simulink model "Design_of_an_Energy_Efficient_Hybrid_Electric_Vehicle"  (R2023a)
settings: Solver=FixedStepDiscrete  StartTime=0  StopTime=110  RelTol=1e-3  EnableMultiTasking=on
PreLoadFcn:
  | power_motordrive_IPMSM_FOC_data
InitFcn:
  | power_motordrive_IPMSM_FOC_data
  | Cdc  = 0.001;      % DC-link capacitor  [F]
  | AH0  = 280;        % Initial battery charge [hr*A]
  | Tmax=410;
  | 
  | %% Vehicle Parameters for Vehicle Dynamics 2
  | vehicle_mass = 2111;
  | wheel_radius = 0.228;
  | area =2.22;
  | drag_coefficient = 0.23;
  | air_density = 1.204;
  | gravity = 9.81;
  | rolling_res_ratio = 0.02;
  | 
  | % Differential drive parameters
  | gear_ratio = 5;
  | i_t   = gear_ratio ;
  | Rw=wheel_radius;
  | 
  | 
  | %% Sliding Mode Observer
  | pmsm.N_max=wmax;
  | pmsm.p=p
  | pmsm.Ld=Ld;
  | pmsm.Lq=Lq;
  | pmsm.Rs=Rs;
  | PU_System.V_base=(Vdc_nom/sqrt(3));
  | PU_System.I_base=lambda/(Lq-Ld);
  | max_torque=400
  | force_max_pedal=500
  | braking_torque_to_pedal_force_ratio=-4
undefined symbols (not defined in the file): BlkSampleTime, CurrentObserverGain, dataType, DiscIntNeverNeededParam, Fsw, gcbh, Ki_Ireg, Ki_wreg, Kp_Ireg, Kp_wreg, L_smo_gain, lambda, Ld, Limit_Ireg, Limit_wreg, Lq, MaxApplicationSpeed, MaxStatorCurrent, MaxStatorVoltage, NumBits1, NumBits2, p, Pmsm, PolePairs, QPLL, rpm_data, Sensorless, sigbuilder_block, SlidingLimit, Slope1, Slope2, sps_rtmsupport, StatorInductance, StatorResistance, Tmax_data, Tnom, Ts, Vdc_nom, wmax
libraries: fl_lib x27, nesl_utility x24, simulink x23, mcbcontrolslib x15, fl_ps_legacy_lib x9, spsStairGeneratorLib x7, sdl_lib x6, ee_lib x4, mcbpositiondecoderlib x4, BoomBox x3, tiiqmathlib x2, autolibshared x2
(part 2 of 4)

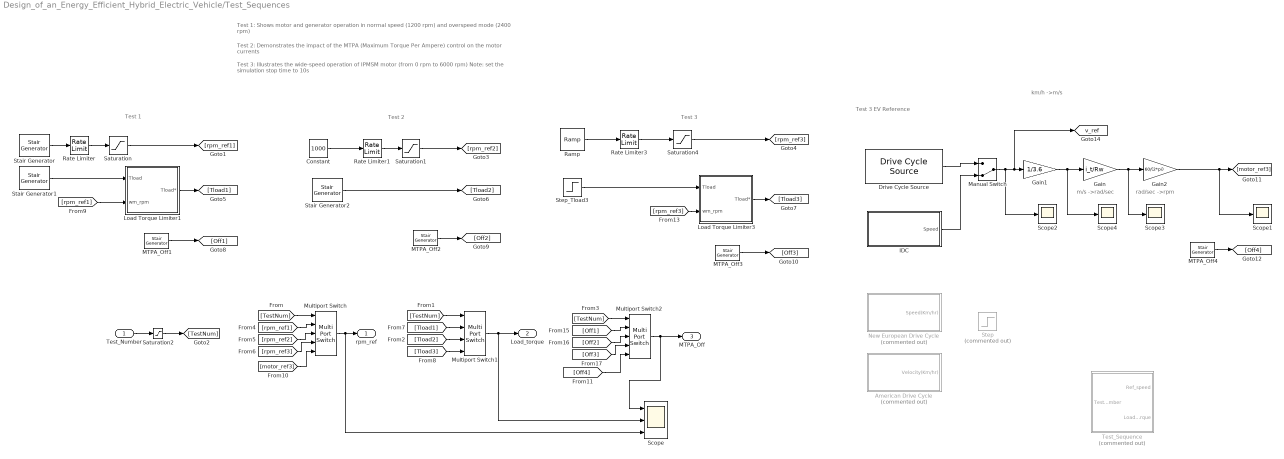
== system Design_of_an_Energy_Efficient_Hybrid_Electric_Vehicle/Test_Sequences ==
  note: Test 1
  note: Test 2
  note: Test 3
  note: Test 1: Shows motor and generator operation in normal speed (1200 rpm) and overspeed mode (2400 rpm)
  note: Test 2: Demonstrates the impact of the MTPA (Maximum Torque Per Ampere) control on the motor currents
  note: Test 3: Illustrates the wide-speed operation of IPMSM motor (from 0 rpm to 6000 rpm)
      | Note: set the simulation stop time to 10s
  note: Test 3 EV Reference
  note: rad/sec ->rpm
  note: m/s ->rad/sec
  note: km/h ->m/s
  Test_Number : Inport
  American Drive Cycle : Subsystem  Tag=STV Subsys  Commented=on  LoadFcn=sigbuilder_block('load');  StartFcn=sigbuilder_block('start');  StopFcn=sigbuilder_block('stop');  ClipboardFcn=sigbuilder_block('clipboard');  mask(Sigbuilder block){tuvar=[0:10]}
      mask help: Simulink:masks:SigbuilderBlock_MD
      mask init:
      | if ~strcmp(get_param(bdroot(gcbh),'SimulationStatus'),'stopped') tuvar = sigbuilder_block('maskInit'); end
      settings: CopyFcn=sigbuilder_block('copy');  DeleteFcn=sigbuilder_block('delete');  ModelCloseFcn=sigbuilder_block('modelClose');  PreSaveFcn=sigbuilder_block('preSave');  PauseFcn=sigbuilder_block('pause');  ContinueFcn=sigbuilder_block('continue');  NameChangeFcn=sigbuilder_block('namechange');  OpenFcn=sigbuilder_block('open',[423.6 162.6 550.8 400.2 ]);  CloseFcn=sigbuilder_block('close');
      mask Display: plot(0, 0, 100, 100,[2, 2, 32, 32, 2], [68, 8, 8, 68, 68],[32, 2], [38, 38], [32, 19, 2],[53, 60, 44], [32, 17, 17, 2],[16, 16, 31, 31]);txt = getActiveGroup(gcbh);text(2, 100, txt,'verticalAlignment', 'top');
  Constant : Constant  Value=1000
  Drive Cycle Source : autolibshared/Drive Cycle Source  cycleVar=FTP75  fileVar=cycleFTP75.mat  tfinal="2474  seconds"  cycleRepeat=off  outAccPort=off  outGearPort=off  gearList=No gear data  t_wot1=5  xdot_woto=0  xdot_wot1=30  t_wot2=20  xdot_wot2=0  t_wotend=30  srcUnit=m/s  outUnit=km/h  srcAccUnit=m/s/s  outAccUnit=m/s^2  dt=0  aMode=1  faultOption=off  velBnd=2  velBndUnit=mph  inUnit=m/s  timeBnd=1  failOption=off  stopSim=off  maxFaultCnt=10  maxFaultTime=2  maxTotFaultTime=15  traceOption=off  dtTrace=1  traceWindow=10  lastDCname=FTP75  lastOutUnit=mph  lastDT=0  lastTB=1  lastSB=2  forceCalcBound=off
  Gain : Gain  Gain=i_t/Rw
  Gain1 : Gain  Gain=1/3.6
  Gain2 : Gain  Gain=60/(2*pi)
  IDC : Subsystem  Tag=STV Subsys  LoadFcn=sigbuilder_block('load');  StartFcn=sigbuilder_block('start');  StopFcn=sigbuilder_block('stop');  ClipboardFcn=sigbuilder_block('clipboard');  mask(Sigbuilder block){tuvar=[0:10]}
      mask help: Simulink:masks:SigbuilderBlock_MD
      mask init:
      | if ~strcmp(get_param(bdroot(gcbh),'SimulationStatus'),'stopped') tuvar = sigbuilder_block('maskInit'); end
      settings: CopyFcn=sigbuilder_block('copy');  DeleteFcn=sigbuilder_block('delete');  ModelCloseFcn=sigbuilder_block('modelClose');  PreSaveFcn=sigbuilder_block('preSave');  PauseFcn=sigbuilder_block('pause');  ContinueFcn=sigbuilder_block('continue');  NameChangeFcn=sigbuilder_block('namechange');  OpenFcn=sigbuilder_block('open',[441 202.5 577.5 270 ]);  CloseFcn=sigbuilder_block('close');
      mask Display: plot(0, 0, 100, 100,[2, 2, 32, 32, 2], [68, 8, 8, 68, 68],[32, 2], [38, 38], [32, 19, 2],[53, 60, 44], [32, 17, 17, 2],[16, 16, 31, 31]);txt = getActiveGroup(gcbh);text(2, 100, txt,'verticalAlignment', 'top');
  Load Torque Limiter1 : Subsystem
  Load Torque Limiter3 : Subsystem
  MTPA_Off1 : spsStairGeneratorLib/Stair Generator  t=[0, 0.9]  e=[0, 1]*0  Ts=Ts
  MTPA_Off2 : spsStairGeneratorLib/Stair Generator  t=[0, 0.8]  e=[0, 1]  Ts=Ts
  MTPA_Off3 : spsStairGeneratorLib/Stair Generator  t=[0, 1.8]  e=[0, 1]*0  Ts=Ts
  MTPA_Off4 : spsStairGeneratorLib/Stair Generator  t=[0, 1.8]  e=[0, 1]*0  Ts=Ts
  Manual Switch : ManualSwitch  CurrentSetting=0
  Multiport Switch : MultiPortSwitch  Inputs=4  SaturateOnIntegerOverflow=off  InputSameDT=off
  Multiport Switch1 : MultiPortSwitch  SaturateOnIntegerOverflow=off  InputSameDT=off
  Multiport Switch2 : MultiPortSwitch  Inputs=4  SaturateOnIntegerOverflow=off  InputSameDT=off
  New European Drive Cycle : Subsystem  Tag=STV Subsys  Commented=on  LoadFcn=sigbuilder_block('load');  StartFcn=sigbuilder_block('start');  StopFcn=sigbuilder_block('stop');  ClipboardFcn=sigbuilder_block('clipboard');  mask(Sigbuilder block){tuvar=[0:10]}
      mask help: Simulink:masks:SigbuilderBlock_MD
      mask init:
      | if ~strcmp(get_param(bdroot(gcbh),'SimulationStatus'),'stopped') tuvar = sigbuilder_block('maskInit'); end
      settings: CopyFcn=sigbuilder_block('copy');  DeleteFcn=sigbuilder_block('delete');  ModelCloseFcn=sigbuilder_block('modelClose');  PreSaveFcn=sigbuilder_block('preSave');  PauseFcn=sigbuilder_block('pause');  ContinueFcn=sigbuilder_block('continue');  NameChangeFcn=sigbuilder_block('namechange');  OpenFcn=sigbuilder_block('open',[75.6 -6 550.8 400.2 ]);  CloseFcn=sigbuilder_block('close');
      mask Display: plot(0, 0, 100, 100,[2, 2, 32, 32, 2], [68, 8, 8, 68, 68],[32, 2], [38, 38], [32, 19, 2],[53, 60, 44], [32, 17, 17, 2],[16, 16, 31, 31]);txt = getActiveGroup(gcbh);text(2, 100, txt,'verticalAlignment', 'top');
  Ramp : simulink/Sources/Ramp  slope=1000*0.7  start=0.5  InitialOutput=0
  Rate Limiter : RateLimiter  RisingSlewLimit=8000  FallingSlewLimit=-8000  SampleTimeMode=inherited
  Rate Limiter1 : RateLimiter  RisingSlewLimit=10000  FallingSlewLimit=-10000  SampleTimeMode=inherited
  Rate Limiter3 : RateLimiter  RisingSlewLimit=5000  FallingSlewLimit=-5000  SampleTimeMode=inherited
  Saturation : Saturate  UpperLimit=wmax  LowerLimit=0
  Saturation1 : Saturate  UpperLimit=wmax  LowerLimit=0
  Saturation2 : Saturate  UpperLimit=4  LowerLimit=1
  Saturation4 : Saturate  UpperLimit=wmax  LowerLimit=0
  Scope : Scope  NumInputPorts=3
  Scope{1..4} (4 alike) : Scope
  Stair Generator : spsStairGeneratorLib/Stair Generator  t=[0,0.7]  e=[1200,2400]  Ts=Ts
  Stair Generator1 : spsStairGeneratorLib/Stair Generator  t="[0,0.4,0.7  1]"  e=[0, 350, 150 -150]  Ts=Ts
  Stair Generator2 : spsStairGeneratorLib/Stair Generator  t=[0,0.4]  e=[0, 350 ]  Ts=Ts
  Step : Step  Commented=on  After=30
  Step_Tload3 : Step  Before=1  After=Tnom  SampleTime=Ts
  Test_Sequence : Subsystem  Commented=on
  rpm_ref : Outport
  Load_torque : Outport  Port=2
  MTPA_Off : Outport  Port=3
  tag scope: v_ref=global
  wires:
  Stair Generator/1 -> Rate Limiter/1
  Rate Limiter/1 -> Saturation/1
  Saturation/1 -> [rpm_ref1]
  Multiport Switch/1 -> Scope/3, rpm_ref/1
  Test_Number/1 -> Saturation2/1
  Saturation2/1 -> [TestNum]
  [TestNum] -> Multiport Switch/1
  Rate Limiter3/1 -> Saturation4/1
  Saturation4/1 -> [rpm_ref3]
  [rpm_ref1] -> Multiport Switch/2
  [rpm_ref2] -> Multiport Switch/3
  [rpm_ref3] -> Multiport Switch/4
  [Tload3] -> Multiport Switch1/4
  [Tload2] -> Multiport Switch1/3
  [Tload1] -> Multiport Switch1/2
  [TestNum] -> Multiport Switch1/1
  Multiport Switch1/1 -> Scope/2, Load_torque/1
  Load Torque Limiter3/1(Tload*) -> [Tload3]
  Multiport Switch2/1 -> Scope/1, MTPA_Off/1
  [TestNum] -> Multiport Switch2/1
  [Off1] -> Multiport Switch2/2
  [Off2] -> Multiport Switch2/3
  [Off3] -> Multiport Switch2/4
  MTPA_Off1/1 -> [Off1]
  MTPA_Off2/1 -> [Off2]
  MTPA_Off3/1 -> [Off3]
  Saturation1/1 -> [rpm_ref2]
  Rate Limiter1/1 -> Saturation1/1
  Constant/1 -> Rate Limiter1/1
  Ramp/1 -> Rate Limiter3/1
  [rpm_ref3] -> Load Torque Limiter3/2(wm_rpm)
  [rpm_ref1] -> Load Torque Limiter1/2(wm_rpm)
  Load Torque Limiter1/1(Tload*) -> [Tload1]
  Step_Tload3/1 -> Load Torque Limiter3/1(Tload)
  Stair Generator1/1 -> Load Torque Limiter1/1(Tload)
  Stair Generator2/1 -> [Tload2]
  Drive Cycle Source/1 -> Manual Switch/1
  Gain1/1 -> Scope4/1, Gain/1
  Gain2/1 -> Scope1/1, [motor_ref3]
  Gain/1 -> Scope3/1, Gain2/1
  [motor_ref3] -> Multiport Switch/5
  MTPA_Off4/1 -> [Off4]
  [Off4] -> Multiport Switch2/5
  Manual Switch/1 -> Scope2/1, [v_ref], Gain1/1
  IDC/1(Speed) -> Manual Switch/2

== system Design_of_an_Energy_Efficient_Hybrid_Electric_Vehicle/Vehicle Controller ==
  Acc : Inport
  Brk : Inport  Port=2
  Rate Transition : RateTransition
  Rate Transition1 : RateTransition
  Rate Transition2 : RateTransition
  Task_10ms : simulink/Ports & Subsystems/Function-Call Generator  sample_time=0.01  numberOfIterations=1  DisallowWideOutput=off
  Vehicle Controller : Subsystem
  trqR : Outport  VectorParamsAs1DForOutWhenUnconnected=off
  tag scope: Acceleration=global, Brake=global
  wires:
  Acc/1 -> Rate Transition/1
  Task_10ms/1 -> Vehicle Controller/Trigger
  Vehicle Controller/1(TqRequest) -> trqR/1
  Brk/1 -> Rate Transition1/1
  Rate Transition/1 -> Vehicle Controller/1(AccPedal [0,1]), [Acceleration]
  Rate Transition1/1 -> [Brake], Vehicle Controller/2(BrakePedal [0,1])
  [v] -> Rate Transition2/1
  Rate Transition2/1 -> Vehicle Controller/3(v [km/h])

== system Design_of_an_Energy_Efficient_Hybrid_Electric_Vehicle/All-Terrain Vehicle Model/Brake Torque ==
  Pedal : Inport
  Dead Zone : DeadZone  LowerValue=-Tmax*i_t  UpperValue=Tmax*i_t
  Force for max pedal deflection : Gain  Gain=force_max_pedal
  Ideal Torque Source : fl_lib/Mechanical/Mechanical Sources/Ideal Torque Source
  MRRef : fl_lib/Mechanical/Rotational Elements/Mechanical Rotational Reference
  Motion Sensor : fl_lib/Mechanical/Mechanical Sensors/Ideal Rotational Motion Sensor  reference=foundation.enum.MeasurementReference.difference  acceleration_port=false  velocity_port=true  position_port=true  wrap_angle=simscape.enum.onoff.off  offset=0 rad
  PS Product : fl_ps_legacy_lib/Legacy Physical Signals/Functions/PS Product
  Scope : Scope
  Scope1 : Scope
  Scope2 : Scope
  Simulink-PS Converter1 : nesl_utility/Simulink-PS Converter  PhysicalDomain=network_engine_domain  SubClassName=ps_input  LeftPortType=input  RightPortType=output  PseudoPeriodic=off  Frequencies=[]  NoiseDistribution=none  NoiseParameters=[]  Unit=N*m  AffineConversion=off  FilteringAndDerivatives=zero  SimscapeFilterOrder=1  InputFilterTimeConstant=0.001  UdotUserProvided=1
  Smooth Sign : Subsystem
  Torque per unit brake pedal force : Gain  Gain=braking_torque_to_pedal_force_ratio
  R : PMIOPort  Side=Right
  wires:
  Pedal/1 -> Force for max pedal deflection/1
  Force for max pedal deflection/1 -> Scope2/1, Torque per unit brake pedal force/1
  Torque per unit brake pedal force/1 -> Scope/1, Dead Zone/1
  Dead Zone/1 -> Scope1/1, Simulink-PS Converter1/1
  connections:
  Smooth Sign/RConn1 -- PS Product/LConn2
  Motion Sensor/RConn1 -- MRRef/LConn1 -- Ideal Torque Source/RConn2
  Ideal Torque Source/LConn1 -- Motion Sensor/LConn1 -- R/RConn1
  PS Product/RConn1 -- Ideal Torque Source/RConn1
  Simulink-PS Converter1/RConn1 -- PS Product/LConn1
  Smooth Sign/LConn1 -- Motion Sensor/RConn2

== system Design_of_an_Energy_Efficient_Hybrid_Electric_Vehicle/All-Terrain Vehicle Model/Sensor Subsystem ==
  Ideal Translational Motion Sensor : fl_lib/Mechanical/Mechanical Sensors/Ideal Translational Motion Sensor  reference=foundation.enum.MeasurementReference.difference  acceleration_port=false  velocity_port=true  position_port=true  offset=0 m
  Mechanical Translational Reference : fl_lib/Mechanical/Translational Elements/Mechanical Translational Reference
  PS-Simulink Converter1 : nesl_utility/PS-Simulink Converter  PhysicalDomain=network_engine_domain  SubClassName=ps_output  LeftPortType=input  RightPortType=output  PseudoPeriodic=off  Frequencies=[]  VectorFormat=1-D array  Unit=km/hr  AffineConversion=off
  PS-Simulink Converter2 : nesl_utility/PS-Simulink Converter  PhysicalDomain=network_engine_domain  SubClassName=ps_output  LeftPortType=input  RightPortType=output  PseudoPeriodic=off  Frequencies=[]  VectorFormat=1-D array  Unit=1  AffineConversion=off
  PS-Simulink Converter3 : nesl_utility/PS-Simulink Converter  PhysicalDomain=network_engine_domain  SubClassName=ps_output  LeftPortType=input  RightPortType=output  PseudoPeriodic=off  Frequencies=[]  VectorFormat=1-D array  Unit=mph  AffineConversion=off
  Vehicle : PMIOPort  Side=Left
  Pos : PMIOPort  Port=2  Side=Right
  mph : Outport  VectorParamsAs1DForOutWhenUnconnected=off
  kmph : Outport  Port=2  VectorParamsAs1DForOutWhenUnconnected=off
  m : Outport  Port=3  VectorParamsAs1DForOutWhenUnconnected=off
  wires:
  PS-Simulink Converter1/1 -> kmph/1
  PS-Simulink Converter2/1 -> m/1
  PS-Simulink Converter3/1 -> mph/1
  connections:
  Mechanical Translational Reference/LConn1 -- Ideal Translational Motion Sensor/RConn1
  PS-Simulink Converter2/LConn1 -- Pos/RConn1 -- Ideal Translational Motion Sensor/RConn3
  Ideal Translational Motion Sensor/RConn2 -- PS-Simulink Converter3/LConn1 -- PS-Simulink Converter1/LConn1
  Ideal Translational Motion Sensor/LConn1 -- Vehicle/RConn1

== system Design_of_an_Energy_Efficient_Hybrid_Electric_Vehicle/Electric Drive/Gate Driver ==
  S : Inport
  Demux : Demux  Outputs=6
  Simulink-PS Converter{1..6} (6 alike) : nesl_utility/Simulink-PS Converter  PhysicalDomain=network_engine_domain  SubClassName=ps_input  LeftPortType=input  RightPortType=output  PseudoPeriodic=off  Frequencies=[]  NoiseDistribution=none  NoiseParameters=[]  Unit=1  AffineConversion=off  FilteringAndDerivatives=zero  SimscapeFilterOrder=1  InputFilterTimeConstant=0.001  UdotUserProvided=1
  Six-Pulse Gate Multiplexer : ee_lib/Semiconductors & Converters/Converters/Six-Pulse Gate Multiplexer  port_option=ee.enum.controlport.ps
  G : PMIOPort  Side=Right
  wires:
  Demux/1 -> Simulink-PS Converter1/1
  S/1 -> Demux/1
  Demux/4 -> Simulink-PS Converter4/1
  Demux/2 -> Simulink-PS Converter2/1
  Demux/3 -> Simulink-PS Converter3/1
  Demux/5 -> Simulink-PS Converter5/1
  Demux/6 -> Simulink-PS Converter6/1
  connections:
  Six-Pulse Gate Multiplexer/RConn1 -- G/RConn1
  Simulink-PS Converter1/RConn1 -- Six-Pulse Gate Multiplexer/LConn1
  Simulink-PS Converter3/RConn1 -- Six-Pulse Gate Multiplexer/LConn3
  Simulink-PS Converter5/RConn1 -- Six-Pulse Gate Multiplexer/LConn5
  Simulink-PS Converter6/RConn1 -- Six-Pulse Gate Multiplexer/LConn6
  Simulink-PS Converter4/RConn1 -- Six-Pulse Gate Multiplexer/LConn4
  Simulink-PS Converter2/RConn1 -- Six-Pulse Gate Multiplexer/LConn2

== system Design_of_an_Energy_Efficient_Hybrid_Electric_Vehicle/Electric Drive/Meas I ==
  Current Sensor : ee_lib/Sensors & Transducers/Current Sensor (Three-Phase)
  PS-Simulink Converter : nesl_utility/PS-Simulink Converter  PhysicalDomain=network_engine_domain  SubClassName=ps_output  LeftPortType=input  RightPortType=output  PseudoPeriodic=off  Frequencies=[]  VectorFormat=1-D array  Unit=A  AffineConversion=off
  1 : PMIOPort  Side=Left
  2 : PMIOPort  Port=2  Side=Right
  iabc : Outport  VectorParamsAs1DForOutWhenUnconnected=off
  tag scope: I_ABC=global
  wires:
  PS-Simulink Converter/1 -> [I_ABC], iabc/1
  connections:
  1/RConn1 -- Current Sensor/LConn1
  2/RConn1 -- Current Sensor/RConn2
  Current Sensor/RConn1 -- PS-Simulink Converter/LConn1

== system Design_of_an_Energy_Efficient_Hybrid_Electric_Vehicle/Electric Drive/Meas V ==
  PS-Simulink Converter4 : nesl_utility/PS-Simulink Converter  PhysicalDomain=network_engine_domain  SubClassName=ps_output  LeftPortType=input  RightPortType=output  PseudoPeriodic=off  Frequencies=[]  VectorFormat=1-D array  Unit=V  AffineConversion=off
  Voltage Sensor : fl_lib/Electrical/Electrical Sensors/Voltage Sensor
  - : PMIOPort  Side=Right
  + : PMIOPort  Port=2  Side=Left
  Vdc : Outport  VectorParamsAs1DForOutWhenUnconnected=off
  wires:
  PS-Simulink Converter4/1 -> Vdc/1
  connections:
  PS-Simulink Converter4/LConn1 -- Voltage Sensor/RConn1
  Voltage Sensor/LConn1 -- +/RConn1
  Voltage Sensor/RConn2 -- -/RConn1

== system Design_of_an_Energy_Efficient_Hybrid_Electric_Vehicle/Electric Drive/Sensor ==
  Display : Display
  Gain : Gain  Gain=30/pi
  MRRef : fl_lib/Mechanical/Rotational Elements/Mechanical Rotational Reference
  Motion Sensor : fl_lib/Mechanical/Mechanical Sensors/Ideal Rotational Motion Sensor  reference=foundation.enum.MeasurementReference.difference  acceleration_port=false  velocity_port=true  position_port=true  wrap_angle=simscape.enum.onoff.off  offset=0 deg
  PS-Simulink Converter1 : nesl_utility/PS-Simulink Converter  PhysicalDomain=network_engine_domain  SubClassName=ps_output  LeftPortType=input  RightPortType=output  PseudoPeriodic=off  Frequencies=[]  VectorFormat=1-D array  Unit=rad/s  AffineConversion=off
  PS-Simulink Converter2 : nesl_utility/PS-Simulink Converter  PhysicalDomain=network_engine_domain  SubClassName=ps_output  LeftPortType=input  RightPortType=output  PseudoPeriodic=off  Frequencies=[]  VectorFormat=1-D array  Unit=rad  AffineConversion=off
  PS-Simulink Converter3 : nesl_utility/PS-Simulink Converter  PhysicalDomain=network_engine_domain  SubClassName=ps_output  LeftPortType=input  RightPortType=output  PseudoPeriodic=off  Frequencies=[]  VectorFormat=1-D array  Unit=N*m  AffineConversion=off
  Scope : Scope
  Scope1 : Scope
  Torque Sensor : fl_lib/Mechanical/Mechanical Sensors/Ideal Torque Sensor
  R : PMIOPort  Side=Left
  C : PMIOPort  Port=2  Side=Right
  w : Outport  VectorParamsAs1DForOutWhenUnconnected=off
  A : Outport  Port=2  VectorParamsAs1DForOutWhenUnconnected=off
  tag scope: Tq_meas=global
  wires:
  PS-Simulink Converter1/1 -> Gain/1, w/1
  PS-Simulink Converter2/1 -> A/1
  PS-Simulink Converter3/1 -> Scope/1, [Tq_meas]
  Gain/1 -> Display/1, Scope1/1
  connections:
  Motion Sensor/RConn2 -- PS-Simulink Converter1/LConn1
  Motion Sensor/RConn1 -- MRRef/LConn1
  R/RConn1 -- Torque Sensor/LConn1
  Torque Sensor/RConn1 -- C/RConn1 -- Motion Sensor/LConn1
  Torque Sensor/RConn2 -- PS-Simulink Converter3/LConn1
  Motion Sensor/RConn3 -- PS-Simulink Converter2/LConn1

== system Design_of_an_Energy_Efficient_Hybrid_Electric_Vehicle/FOC/Alpha&Beta Current Estimation ==
  theta : Inport
  Idq_ref : Inport  Port=2
  Alpha_Beta_Estimation : Subsystem
  Scope6 : Scope
  Transfrom_Alpha_Beta_Estimation : Subsystem
  Ialpha_est : Outport
  Ibeta_est : Outport  Port=2
  "Ialpha\"_est" : Outport  Port=3
  "Ibeta\"_est" : Outport  Port=4
  wires:
  Alpha_Beta_Estimation/1(Ialpha_est) -> Ialpha_est/1
  Idq_ref/1 -> Scope6/1, Alpha_Beta_Estimation/1(Idq_ref), Transfrom_Alpha_Beta_Estimation/1(Idq_ref)
  theta/1 -> Transfrom_Alpha_Beta_Estimation/2(theta), Alpha_Beta_Estimation/2(Theta)
  Alpha_Beta_Estimation/2(Ibeta_est) -> Ibeta_est/1
  Transfrom_Alpha_Beta_Estimation/1("Ialpha\"_est") -> "Ialpha\"_est"/1
  Transfrom_Alpha_Beta_Estimation/2("Ibeta\"_est") -> "Ibeta\"_est"/1

== system Design_of_an_Energy_Efficient_Hybrid_Electric_Vehicle/FOC/Axis Transformation ==
  a : Inport
  b : Inport  Port=2
  -one_by_sqrt3 : Gain  Gain=-1/sqrt(3)  RndMeth=Simplest  OutDataTypeStr=Inherit: Same as input
  a_plus_2b : Sum  Inputs=+++  RndMeth=Simplest  OutDataTypeStr=Inherit: Same as first input
  "Alpha\"" : Outport  VectorParamsAs1DForOutWhenUnconnected=off
  "Beta\"" : Outport  Port=2  VectorParamsAs1DForOutWhenUnconnected=off
  wires:
  a_plus_2b/1 -> -one_by_sqrt3/1
  b/1 -> "Alpha\""/1, a_plus_2b/3
  -one_by_sqrt3/1 -> "Beta\""/1
  a/1 -> a_plus_2b/2, a_plus_2b/1

== system Design_of_an_Energy_Efficient_Hybrid_Electric_Vehicle/FOC/Current reference calculation ==
  Tref : Inport
  wm : Inport  Port=2
  Abs : Abs  SaturateOnIntegerOverflow=off
  Gain1 : Gain  Gain=pi/30
  Gain2 : Gain  Gain=1/Teb  SaturateOnIntegerOverflow=on  OutDataTypeStr=Inherit: Same as input  ParamDataTypeStr=Inherit: Same as input
  Gain3 : Gain  Gain=ib  SaturateOnIntegerOverflow=on  OutDataTypeStr=Inherit: Same as input  ParamDataTypeStr=Inherit: Same as input
  Gain4 : Gain  Gain=ib  SaturateOnIntegerOverflow=on  OutDataTypeStr=Inherit: Same as input  ParamDataTypeStr=Inherit: Same as input
  Ld Lq lam p ib : Constant  Value=[Ld, Lq, lam, p, lam/(Lq-Ld)]
  Ld Lq lam p ib1 : Constant  Value=lam/(Lq-Ld)
  MTPA Field Weakening Controller : MATLAB Function  TreatAsAtomicUnit=on  SystemSampleTime=Ts
  Mux : Mux  Inputs=2
  Optimal iqn : Lookup  InputValues=ten  Table=iqn  SaturateOnIntegerOverflow=off
  Rate Limiter1 : RateLimiter  RisingSlewLimit=20  FallingSlewLimit=-20  SampleTimeMode=inherited
  Rate Limiter4 : RateLimiter  RisingSlewLimit=20*5  FallingSlewLimit=-20*5  SampleTimeMode=inherited
  Scope : Scope
  Vdc : Constant  Value=Vdc_nom
  IdIq_ref : Outport
  wires:
  Mux/1 -> IdIq_ref/1
  Gain3/1 -> Mux/2
  Gain4/1 -> Mux/1
  Tref/1 -> Gain2/1
  Gain2/1 -> Abs/1, MTPA Field Weakening Controller/2(Ten)  "Ten"
  wm/1 -> Gain1/1
  Ld Lq lam p ib/1 -> MTPA Field Weakening Controller/5(params)
  Optimal iqn/1 -> MTPA Field Weakening Controller/1(iqn_opt)
  Abs/1 -> Optimal iqn/1
  Vdc/1 -> MTPA Field Weakening Controller/4(Vdc)
  Gain1/1 -> MTPA Field Weakening Controller/3(w)
  MTPA Field Weakening Controller/1(iqn) -> Rate Limiter4/1
  MTPA Field Weakening Controller/2(idn) -> Rate Limiter1/1
  Rate Limiter1/1 -> Gain4/1
  Rate Limiter4/1 -> Gain3/1
  Ld Lq lam p ib1/1 -> Scope/1

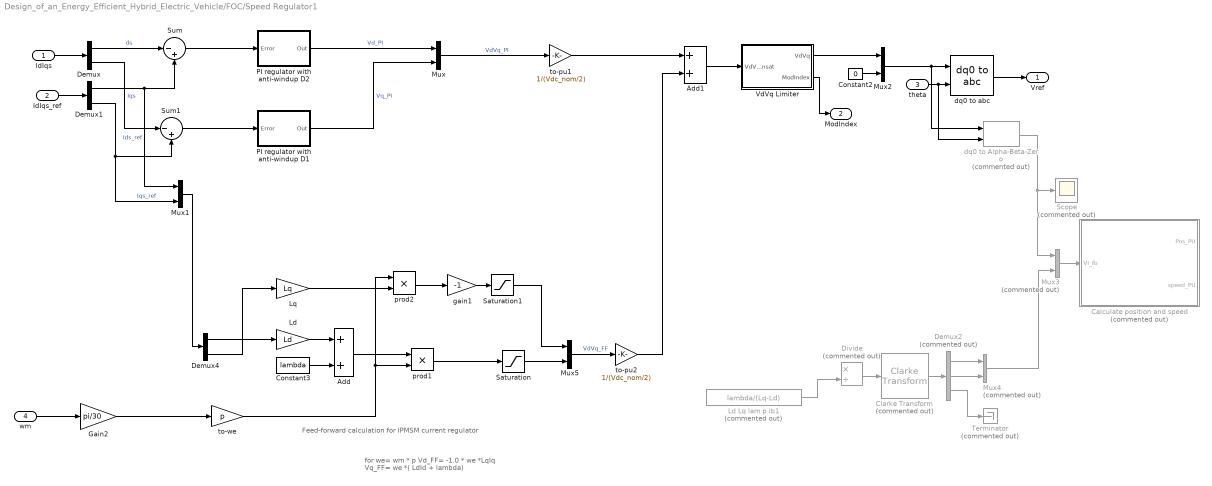
== system Design_of_an_Energy_Efficient_Hybrid_Electric_Vehicle/FOC/Speed Regulator1 ==
  note: for we= wm * p
      | Vd_FF= -1.0 * we *LqIq
      | Vq_FF= we *( LdId + lambda)
  note: Feed-forward calculation for IPMSM current regulator
  IdIqs : Inport  PortDimensions=2
  IdIqs_ref : Inport  Port=2  PortDimensions=2
  theta : Inport  Port=3  PortDimensions=1
  wm : Inport  Port=4  PortDimensions=1
  Add : Sum
  Add1 : Sum
  Calculate position and speed : Subsystem  Commented=on
  Clarke Transform : eeTransforms/Clarke Transform  Commented=on  PowerInvariant=off
  Constant2 : Constant  Value=0
  Constant3 : Constant  Value=lambda  OutDataTypeStr=Inherit: Inherit via back propagation  SampleTime=-1
  Demux : Demux  Outputs=2
  Demux1 : Demux  Outputs=2
  Demux2 : Demux  Commented=on  Outputs=3
  Demux4 : Demux  Outputs=2
  Divide : Product  Commented=on  Inputs=*/
  Gain2 : Gain  Gain=pi/30
  Ld : Gain  Gain=Ld  RndMeth=Simplest  OutDataTypeStr=Inherit: Same as input  ParamDataTypeStr=Inherit: Same as input
  Ld Lq lam p ib1 : Constant  Commented=on  Value=lambda/(Lq-Ld)
  Lq : Gain  Gain=Lq  RndMeth=Simplest  OutDataTypeStr=Inherit: Same as input  ParamDataTypeStr=Inherit: Same as input
  Mux : Mux  Inputs=2
  Mux1 : Mux  Inputs=2
  Mux2 : Mux  Inputs=[2,1]
  Mux3 : Mux  Commented=on  Inputs=2
  Mux4 : Mux  Commented=on  Inputs=2
  Mux5 : Mux  Inputs=2
  PI regulator with anti-windup D1 : Subsystem  DialogController=POWERSYS.PowerSysDialog  mask(Discrete PI Controller){Kp=Kp, Ki=Ki, Par_Limits=[Limits -Limits], Init=0, Ts=Ts}
      mask prompts: Kp "Proportional gain (Kp):"; Ki "Integral gain (Ki):"; Par_Limits "Output limits: [ Upper   Lower ]"; Init "Output initial value:"; Ts "Sample time:"
      mask help: This block implements a discrete PI controller.
      mask init:
      | UpperLimit=Par_Limits(1);
      | LowerLimit=Par_Limits(2);
      | power_initmask();
      mask Help: This block is part of a subset of blocks in the Extras library that does not have documentation associated with it, other than the block mask description.
      mask Display: disp('PI');
  PI regulator with anti-windup D2 : Subsystem  DialogController=POWERSYS.PowerSysDialog  mask(Discrete PI Controller){Kp=Kp, Ki=Ki, Par_Limits=[Limits -Limits], Init=0, Ts=Ts}
      mask prompts: Kp "Proportional gain (Kp):"; Ki "Integral gain (Ki):"; Par_Limits "Output limits: [ Upper   Lower ]"; Init "Output initial value:"; Ts "Sample time:"
      mask help: This block implements a discrete PI controller.
      mask init:
      | UpperLimit=Par_Limits(1);
      | LowerLimit=Par_Limits(2);
      | power_initmask();
      mask Help: This block is part of a subset of blocks in the Extras library that does not have documentation associated with it, other than the block mask description.
      mask Display: disp('PI');
  Saturation : Saturate  UpperLimit=Vdc_nom/sqrt(3)  LowerLimit=-Vdc_nom/sqrt(3)  RndMeth=Simplest
  Saturation1 : Saturate  UpperLimit=Vdc_nom/sqrt(3)  LowerLimit=-Vdc_nom/sqrt(3)  RndMeth=Simplest
  Scope : Scope  Commented=on
  Sum : Sum  Inputs=|-+
  Sum1 : Sum  Inputs=|-+
  Terminator : Terminator  Commented=on
  VdVq Limiter : Subsystem
  dq0 to Alpha-Beta-Zero : spsdq0toAlphaBetaZeroLib/dq0 to Alpha-Beta-Zero  Commented=on  Alignment=90 degrees behind phase A axis
  dq0 to abc : spsdq0toabcLib/dq0 to abc  Alignment=90 degrees behind phase A axis
  gain1 : Gain  Gain=-1  RndMeth=Simplest  OutDataTypeStr=Inherit: Same as input  ParamDataTypeStr=Inherit: Same as input
  prod1 : Product  RndMeth=Simplest  OutDataTypeStr=Inherit: Same as first input
  prod2 : Product  RndMeth=Simplest  OutDataTypeStr=Inherit: Same as first input
  to-pu1 : Gain  Gain=1/(Vdc_nom/2)
  to-pu2 : Gain  Gain=1/(Vdc_nom/2)
  to-we : Gain  Gain=p  RndMeth=Simplest  OutDataTypeStr=Inherit: Same as input  ParamDataTypeStr=Inherit: Same as input
  Vref : Outport
  ModIndex : Outport  Port=2
  wires:
  to-pu2/1 -> Add1/2
  to-pu1/1 -> Add1/1
  Demux1/1 -> Mux1/1, Sum/2  "Ids_ref"
  Demux/1 -> Sum/1  "ds"
  Demux1/2 -> Sum1/2, Mux1/2  "Iqs_ref"
  IdIqs_ref/1 -> Demux1/1
  IdIqs/1 -> Demux/1
  Sum/1 -> PI regulator with anti-windup D2/1(Error)
  Sum1/1 -> PI regulator with anti-windup D1/1(Error)
  theta/1 -> dq0 to Alpha-Beta-Zero/2, dq0 to abc/2
  Demux/2 -> Sum1/1  "Iqs"
  dq0 to abc/1 -> Vref/1
  wm/1 -> Gain2/1
  Mux1/1 -> Demux4/1
  PI regulator with anti-windup D2/1(Out) -> Mux/1  "Vd_PI"
  PI regulator with anti-windup D1/1(Out) -> Mux/2  "Vq_PI"
  Mux/1 -> to-pu1/1  "VdVq_PI"
  Mux5/1 -> to-pu2/1  "VdVq_FF"
  Add1/1 -> VdVq Limiter/1(VdVq_unsat)
  VdVq Limiter/1(VdVq) -> Mux2/1
  Constant2/1 -> Mux2/2
  Mux2/1 -> dq0 to Alpha-Beta-Zero/1, dq0 to abc/1
  VdVq Limiter/2(ModIndex) -> ModIndex/1
  Demux4/2 -> Lq/1
  Lq/1 -> prod2/2
  gain1/1 -> Saturation1/1
  Demux4/1 -> Ld/1
  Add/1 -> prod1/1
  to-we/1 -> prod2/1, prod1/2
  Saturation1/1 -> Mux5/1
  prod2/1 -> gain1/1
  Constant3/1 -> Add/2
  Saturation/1 -> Mux5/2
  Ld/1 -> Add/1
  prod1/1 -> Saturation/1
  Gain2/1 -> to-we/1
  dq0 to Alpha-Beta-Zero/1 -> Mux3/1, Scope/1
  Mux3/1 -> Calculate position and speed/1(VI_fb)
  ? -> Divide/1
  Ld Lq lam p ib1/1 -> Divide/2
  Divide/1 -> Clarke Transform/1
  Clarke Transform/1 -> Demux2/1
  Demux2/1 -> Mux4/1
  Demux2/2 -> Mux4/2
  Mux4/1 -> Mux3/2
  Demux2/3 -> Terminator/1

== system Design_of_an_Energy_Efficient_Hybrid_Electric_Vehicle/FOC/Speed Regulator2 ==
  note: Anti-windup mechanism: Method of conditionnal integration
      |
      | The integration is suspended if saturation occurs and the
      | control error is of the same sign as the control signal.
      |
      | [1] L.Rundqwist, "Anti-Reset Windup for PID Controllers," Ph.D. Thesis TRFT-1033,
      | Departement of Automatic Control, Lund Institute of Technology, Lund, Sweeden, 1991.
  wref : Inport  PortDimensions=1
  w : Inport  Port=2  PortDimensions=1
  Add : Sum  Inputs=+|-
  Compare To Zero : simulink/Logic and Bit Operations/Compare To Zero  relop=>  OutDataTypeStr=uint8  ZeroCross=off
  Compare To Zero1 : simulink/Logic and Bit Operations/Compare To Zero  relop=<  OutDataTypeStr=uint8  ZeroCross=off
  Constant : Constant  Value=0
  Constant1 : Constant  Value=Limit_wreg
  Constant2 : Constant  Value=-Limit_wreg
  Discrete-Time Integrator : DiscreteIntegrator  IntegratorMethod=Integration: Trapezoidal  InitialCondition=Init  SampleTime=Ts  LimitOutput=on  UpperSaturationLimit=Limit_wreg  LowerSaturationLimit=-Limit_wreg  ShowStatePort=on  ICPrevOutput=DiscIntNeverNeededParam  ICPrevScaledInput=DiscIntNeverNeededParam
  Kp4 : Gain  Gain=Kp  SaturateOnIntegerOverflow=on  SampleTime=Ts  OutDataTypeStr=Inherit: Same as input  ParamDataTypeStr=Inherit: Same as input
  Kp5 : Gain  Gain=Ki  SaturateOnIntegerOverflow=on  SampleTime=Ts  OutDataTypeStr=Inherit: Same as input  ParamDataTypeStr=Inherit: Same as input
  Logical Operator : Logic  AllPortsSameDT=off  OutDataTypeStr=boolean
  Logical Operator1 : Logic  AllPortsSameDT=off  OutDataTypeStr=boolean
  Logical Operator2 : Logic  Operator=OR  AllPortsSameDT=off  OutDataTypeStr=boolean
  Relational Operator : RelationalOperator  OutDataTypeStr=boolean  InputSameDT=off
  Relational Operator1 : RelationalOperator  Operator=<=  OutDataTypeStr=boolean  InputSameDT=off
  Saturation2 : Saturate  UpperLimit=Limit_wreg  LowerLimit=-Limit_wreg  SampleTime=Ts
  Sum1 : Sum  InputSameDT=on  SaturateOnIntegerOverflow=on  SampleTime=Ts  OutDataTypeStr=Inherit: Same as first input
  Sum6 : Sum  InputSameDT=on  SaturateOnIntegerOverflow=on  SampleTime=Ts  OutDataTypeStr=Inherit: Same as first input
  Switch : Switch  Criteria=u2 > Threshold  SaturateOnIntegerOverflow=off  InputSameDT=off
  Zero-Order Hold : ZeroOrderHold  SampleTime=Ts
  Tref : Outport  SampleTime=Ts  InitialOutput=0  VectorParamsAs1DForOutWhenUnconnected=off
  wires:
  w/1 -> Add/2
  wref/1 -> Add/1
  Constant/1 -> Switch/1
  Zero-Order Hold/1 -> Sum1/2, Sum6/1
  Discrete-Time Integrator/State -> Sum1/1
  Sum1/1 -> Relational Operator1/1, Relational Operator/1
  Logical Operator2/1 -> Switch/2
  Relational Operator/1 -> Logical Operator/1  "UpperLimit_is_Reached"
  Relational Operator1/1 -> Logical Operator1/1  "LowerLimit_Is_Reached"
  Constant1/1 -> Relational Operator/2
  Constant2/1 -> Relational Operator1/2
  Compare To Zero/1 -> Logical Operator/2  "Error_is_positive"
  Logical Operator/1 -> Logical Operator2/1
  Logical Operator1/1 -> Logical Operator2/2
  Compare To Zero1/1 -> Logical Operator1/2  "Error_is_negative"
  Add/1 -> Kp4/1, Kp5/1, Compare To Zero1/1, Compare To Zero/1
  Sum6/1 -> Saturation2/1
  Kp4/1 -> Zero-Order Hold/1
  Discrete-Time Integrator/1 -> Sum6/2
  Saturation2/1 -> Tref/1
  Switch/1 -> Discrete-Time Integrator/1
  Kp5/1 -> Switch/3

== system Design_of_an_Energy_Efficient_Hybrid_Electric_Vehicle/FOC/Torque limiter ==
  Tref : Inport
  wm_rpm : Inport  Port=2
  Abs1 : Abs
  Gain : Gain  Gain=-1
  Saturation Dynamic : simulink/Discontinuities/Saturation Dynamic  OutMin=[]  OutMax=[]  OutDataTypeStr=Inherit: Same as second input  OutDataType=sfix(16)  OutScaling=2^-10  DoSatur=off
  Torque vs speed profile1 : Lookup  InputValues=rpm_data  Table=Tmax_data  SaturateOnIntegerOverflow=off
  Tref* : Outport  VectorParamsAs1DForOutWhenUnconnected=off
  wires:
  wm_rpm/1 -> Abs1/1
  Abs1/1 -> Torque vs speed profile1/1
  Torque vs speed profile1/1 -> Saturation Dynamic/1, Gain/1
  Saturation Dynamic/1 -> Tref*/1
  Tref/1 -> Saturation Dynamic/2
  Gain/1 -> Saturation Dynamic/3

== system Design_of_an_Energy_Efficient_Hybrid_Electric_Vehicle/Test_Sequences/American Drive Cycle ==
  Demux : Demux  Tag=STV Demux  Outputs=1
      settings: DisplayOption=none
  FromWs : FromWorkspace  Tag=STV FromWs  VariableName=tuvar
      SigBuilderData=|
      | common.afterFinalStr = 'Extrapolate'
      | common.sampleTime = 0
      | dataSet.timeRange = [0 600]
      | dataSet.name = 'Sheet1'
      | sbobj.Groups.Name = 'Sheet1'
      | sbobj.Groups.Signals.Name = 'Velocity(Km/hr)'
      | sbobj.Groups.Signals.XData = [0 9 30 36 48 54 66 72 78 84 90 102 120 126 132 141 150 162 174 186 198 210 288 300 306 312 324 330 342 348 354 360 372 414 447 462 489 498 504 510 516 534 540 552 558 564 582 594 600]
      | sbobj.Groups.Signals.YData = [0 70 62 62 0 0 90 88 88 83.5 83.5 115 55 0 0 80 85 98 86 82 100 105 100 120 117 115 130 120 132 103 105 103 109 115 98 100 0 0 43 10 43 1 40 45 0 0 82 0 0]
      | sbobj.Groups.TimeRange = [0 600]
  Velocity(Km/hr) : Outport  Tag=STV Outport
  wires:
  Demux/1 -> Velocity(Km/hr)/1
  FromWs/1 -> Demux/1

== system Design_of_an_Energy_Efficient_Hybrid_Electric_Vehicle/Test_Sequences/IDC ==
  Demux : Demux  Tag=STV Demux  Outputs=1
      settings: DisplayOption=none
  FromWs : FromWorkspace  Tag=STV FromWs  VariableName=tuvar
      SigBuilderData=|
      | common.afterFinalStr = 'Extrapolate'
      | common.sampleTime = '0'
      | dataSet.timeRange = [0 130]
      | dataSet.name = 'Test 1'
      | sbobj.Groups.Name = 'Test 1'
      | sbobj.Groups.Signals.Name = 'Speed'
      | sbobj.Groups.Signals.XData = [0 17 20 28 30 35 40 50 55 60 75 80 90 120 130]
      | sbobj.Groups.Signals.YData = [0 0 17.5 6 6 30 24 24 41 35.5 35.5 31 40 5 -8.4]
      | sbobj.Groups.TimeRange = [0 130]
  Speed : Outport  Tag=STV Outport  VectorParamsAs1DForOutWhenUnconnected=off
  wires:
  FromWs/1 -> Demux/1
  Demux/1 -> Speed/1

== system Design_of_an_Energy_Efficient_Hybrid_Electric_Vehicle/Test_Sequences/Load Torque Limiter1 ==
  Tload : Inport
  wm_rpm : Inport  Port=2
  Abs1 : Abs
  Gain : Gain  Gain=-1
  Saturation Dynamic : simulink/Discontinuities/Saturation Dynamic  OutMin=[]  OutMax=[]  OutDataTypeStr=Inherit: Same as second input  OutDataType=sfix(16)  OutScaling=2^-10  DoSatur=off
  Torque vs speed profile : Lookup_n-D  NumberOfTableDimensions=1  BreakpointsForDimension1=rpm_data  BeginIndexSearchUsingPreviousIndexResult=on  Table=Tmax_data*0.85  InternalRulePriority=Speed
  Tload* : Outport  VectorParamsAs1DForOutWhenUnconnected=off
  wires:
  wm_rpm/1 -> Abs1/1
  Abs1/1 -> Torque vs speed profile/1
  Torque vs speed profile/1 -> Saturation Dynamic/1, Gain/1
  Saturation Dynamic/1 -> Tload*/1
  Tload/1 -> Saturation Dynamic/2
  Gain/1 -> Saturation Dynamic/3

== system Design_of_an_Energy_Efficient_Hybrid_Electric_Vehicle/Test_Sequences/Load Torque Limiter3 ==
  Tload : Inport
  wm_rpm : Inport  Port=2
  Abs1 : Abs
  Gain : Gain  Gain=-1
  Saturation Dynamic : simulink/Discontinuities/Saturation Dynamic  OutMin=[]  OutMax=[]  OutDataTypeStr=Inherit: Same as second input  OutDataType=sfix(16)  OutScaling=2^-10  DoSatur=off
  Torque vs speed profile : Lookup_n-D  NumberOfTableDimensions=1  BreakpointsForDimension1=rpm_data  BeginIndexSearchUsingPreviousIndexResult=on  Table=Tmax_data*0.9  InternalRulePriority=Speed
  Tload* : Outport  VectorParamsAs1DForOutWhenUnconnected=off
  wires:
  Gain/1 -> Saturation Dynamic/3
  Tload/1 -> Saturation Dynamic/2
  Saturation Dynamic/1 -> Tload*/1
  Torque vs speed profile/1 -> Gain/1, Saturation Dynamic/1
  Abs1/1 -> Torque vs speed profile/1
  wm_rpm/1 -> Abs1/1

== system Design_of_an_Energy_Efficient_Hybrid_Electric_Vehicle/Test_Sequences/New European Drive Cycle ==
  Demux : Demux  Tag=STV Demux  Outputs=1
      settings: DisplayOption=none
  FromWs : FromWorkspace  Tag=STV FromWs  VariableName=tuvar
      SigBuilderData=|
      | common.afterFinalStr = 'Extrapolate'
      | common.sampleTime = 0
      | dataSet.timeRange = [0 400]
      | dataSet.name = 'Sheet1'
      | sbobj.Groups.Name = 'Sheet1'
      | sbobj.Groups.Signals.Name = 'Speed(Km/hr)'
      | sbobj.Groups.Signals.XData = [0 20 60 110 120 190 200 250 280 355 385 400]
      | sbobj.Groups.Signals.YData = [0 0 70 70 50 50 70 70 90 90 0 0]
      | sbobj.Groups.TimeRange = [0 400]
  Speed(Km/hr) : Outport  Tag=STV Outport
  wires:
  Demux/1 -> Speed(Km/hr)/1
  FromWs/1 -> Demux/1

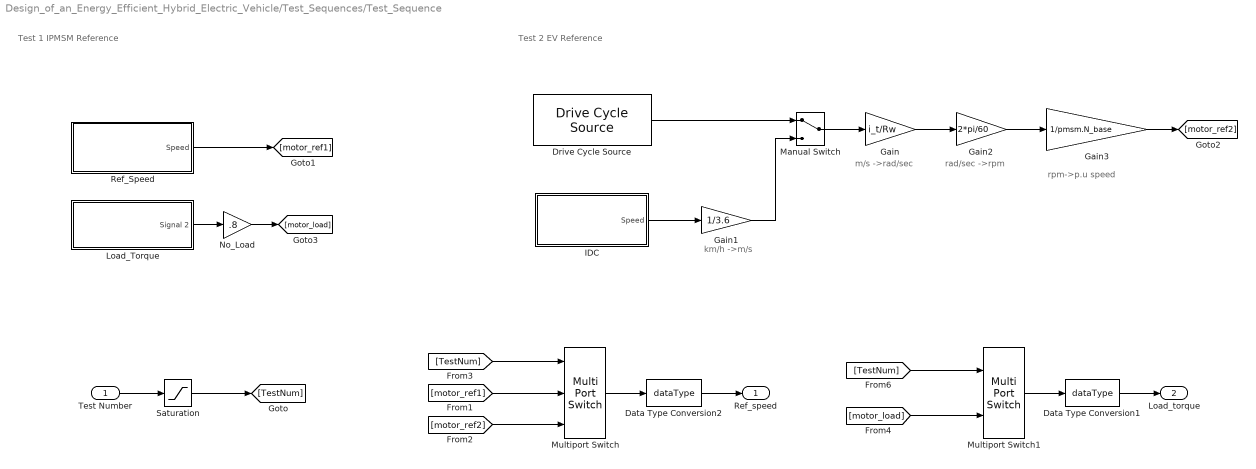
== system Design_of_an_Energy_Efficient_Hybrid_Electric_Vehicle/Test_Sequences/Test_Sequence ==
  note: Test 2 EV Reference
  note: km/h ->m/s
  note: Test 1 IPMSM Reference
  note: m/s ->rad/sec
  note: rad/sec ->rpm
  note: rpm->p.u speed
  Test Number : Inport
  Data Type Conversion1 : DataTypeConversion  OutDataTypeStr=dataType  RndMeth=Simplest  SaturateOnIntegerOverflow=off
  Data Type Conversion2 : DataTypeConversion  OutDataTypeStr=dataType  RndMeth=Simplest  SaturateOnIntegerOverflow=off
  Drive Cycle Source : autolibshared/Drive Cycle Source  cycleVar=EUDC  fileVar=cycleFTP75.mat  tfinal="400  seconds"  cycleRepeat=off  outAccPort=off  outGearPort=off  gearList=No gear data  t_wot1=5  xdot_woto=0  xdot_wot1=30  t_wot2=20  xdot_wot2=0  t_wotend=30  srcUnit=m/s  outUnit=m/s  srcAccUnit=m/s/s  outAccUnit=m/s^2  dt=0  aMode=1  faultOption=off  velBnd=2  velBndUnit=mph  inUnit=m/s  timeBnd=1  failOption=off  stopSim=off  maxFaultCnt=10  maxFaultTime=2  maxTotFaultTime=15  traceOption=off  dtTrace=1  traceWindow=10  lastDCname=EUDC  lastOutUnit=mph  lastDT=0  lastTB=1  lastSB=2  forceCalcBound=off
  Gain : Gain  Gain=i_t/Rw
  Gain1 : Gain  Gain=1/3.6
  Gain2 : Gain  Gain=2*pi/60
  Gain3 : Gain  Gain=1/pmsm.N_base
  IDC : Subsystem  Tag=STV Subsys  LoadFcn=sigbuilder_block('load');  StartFcn=sigbuilder_block('start');  StopFcn=sigbuilder_block('stop');  ClipboardFcn=sigbuilder_block('clipboard');  mask(Sigbuilder block){tuvar=[0:10]}
      mask help: Simulink:masks:SigbuilderBlock_MD
      mask init:
      | if ~strcmp(get_param(bdroot(gcbh),'SimulationStatus'),'stopped') tuvar = sigbuilder_block('maskInit'); end
      settings: CopyFcn=sigbuilder_block('copy');  DeleteFcn=sigbuilder_block('delete');  ModelCloseFcn=sigbuilder_block('modelClose');  PreSaveFcn=sigbuilder_block('preSave');  PauseFcn=sigbuilder_block('pause');  ContinueFcn=sigbuilder_block('continue');  NameChangeFcn=sigbuilder_block('namechange');  OpenFcn=sigbuilder_block('open',[733.5 222 577.5 351 ]);  CloseFcn=sigbuilder_block('close');
      mask Display: plot(0, 0, 100, 100,[2, 2, 32, 32, 2], [68, 8, 8, 68, 68],[32, 2], [38, 38], [32, 19, 2],[53, 60, 44], [32, 17, 17, 2],[16, 16, 31, 31]);txt = getActiveGroup(gcbh);text(2, 100, txt,'verticalAlignment', 'top');
  Load_Torque : Subsystem  Tag=STV Subsys  LoadFcn=sigbuilder_block('load');  StartFcn=sigbuilder_block('start');  StopFcn=sigbuilder_block('stop');  ClipboardFcn=sigbuilder_block('clipboard');  mask(Sigbuilder block){tuvar=[0:10]}
      mask help: Simulink:masks:SigbuilderBlock_MD
      mask init:
      | if ~strcmp(get_param(bdroot(gcbh),'SimulationStatus'),'stopped') tuvar = sigbuilder_block('maskInit'); end
      settings: CopyFcn=sigbuilder_block('copy');  DeleteFcn=sigbuilder_block('delete');  ModelCloseFcn=sigbuilder_block('modelClose');  PreSaveFcn=sigbuilder_block('preSave');  PauseFcn=sigbuilder_block('pause');  ContinueFcn=sigbuilder_block('continue');  NameChangeFcn=sigbuilder_block('namechange');  OpenFcn=sigbuilder_block('open',[474.75 115.5 615 347.25 ]);  CloseFcn=sigbuilder_block('close');
      mask Display: plot(0, 0, 100, 100,[2, 2, 32, 32, 2], [68, 8, 8, 68, 68],[32, 2], [38, 38], [32, 19, 2],[53, 60, 44], [32, 17, 17, 2],[16, 16, 31, 31]);txt = getActiveGroup(gcbh);text(2, 100, txt,'verticalAlignment', 'top');
  Manual Switch : ManualSwitch
  Multiport Switch : MultiPortSwitch  Inputs=2  SaturateOnIntegerOverflow=off  InputSameDT=off
  Multiport Switch1 : MultiPortSwitch  Inputs=1  SaturateOnIntegerOverflow=off  InputSameDT=off
  No_Load : Gain  Gain=.8
  Ref_Speed : Subsystem  Tag=STV Subsys  LoadFcn=sigbuilder_block('load');  StartFcn=sigbuilder_block('start');  StopFcn=sigbuilder_block('stop');  ClipboardFcn=sigbuilder_block('clipboard');  mask(Sigbuilder block){tuvar=[0:10]}
      mask help: Simulink:masks:SigbuilderBlock_MD
      mask init:
      | if ~strcmp(get_param(bdroot(gcbh),'SimulationStatus'),'stopped') tuvar = sigbuilder_block('maskInit'); end
      settings: CopyFcn=sigbuilder_block('copy');  DeleteFcn=sigbuilder_block('delete');  ModelCloseFcn=sigbuilder_block('modelClose');  PreSaveFcn=sigbuilder_block('preSave');  PauseFcn=sigbuilder_block('pause');  ContinueFcn=sigbuilder_block('continue');  NameChangeFcn=sigbuilder_block('namechange');  OpenFcn=sigbuilder_block('open',[856.5 129 577.5 310.5 ]);  CloseFcn=sigbuilder_block('close');
      mask Display: plot(0, 0, 100, 100,[2, 2, 32, 32, 2], [68, 8, 8, 68, 68],[32, 2], [38, 38], [32, 19, 2],[53, 60, 44], [32, 17, 17, 2],[16, 16, 31, 31]);txt = getActiveGroup(gcbh);text(2, 100, txt,'verticalAlignment', 'top');
  Saturation : Saturate  UpperLimit=2  LowerLimit=1
  Ref_speed : Outport
  Load_torque : Outport  Port=2
  wires:
  Test Number/1 -> Saturation/1
  Saturation/1 -> [TestNum]
  Multiport Switch/1 -> Data Type Conversion2/1
  [motor_ref2] -> Multiport Switch/3
  IDC/1(Speed) -> Gain1/1
  Drive Cycle Source/1 -> Manual Switch/1
  Gain1/1 -> Manual Switch/2
  Ref_Speed/1(Speed) -> [motor_ref1]
  [motor_ref1] -> Multiport Switch/2
  Manual Switch/1 -> Gain/1
  [TestNum] -> Multiport Switch/1
  Gain/1 -> Gain2/1
  Gain2/1 -> Gain3/1
  Gain3/1 -> [motor_ref2]
  Data Type Conversion2/1 -> Ref_speed/1
  Load_Torque/1(Signal 2) -> No_Load/1
  No_Load/1 -> [motor_load]
  Multiport Switch1/1 -> Data Type Conversion1/1
  Data Type Conversion1/1 -> Load_torque/1
  [motor_load] -> Multiport Switch1/2
  [TestNum] -> Multiport Switch1/1

== system Design_of_an_Energy_Efficient_Hybrid_Electric_Vehicle/Vehicle Controller/Vehicle Controller ==
  AccPedal [0,1] : Inport
  BrakePedal [0,1] : Inport  Port=2
  v [km/h] : Inport  Port=3
  Task10ms : TriggerPort  TriggerType=function-call  VariantControl=Variant  PortDimensions=1
  Acceleration Pedal Characteristic : Lookup_n-D  NumberOfTableDimensions=1  BreakpointsForDimension1=0:0.1:1  Table=[0 0.04 0.07 0.1 0.16 0.2 0.3 0.4 0.6 0.8 1]*Tmax  InternalRulePriority=Speed  RndMeth=Simplest
  Brake Pedal Characteristic : Lookup_n-D  NumberOfTableDimensions=1  BreakpointsForDimension1=[0 0.03 0.04 0.3 0.4 0.5 0.6 0.7 0.8 0.9 1]  Table=[0 0 0.04 0.05 0.06 0.2 0.25 0.4 0.6 0.8 1]*(-Tmax)  InternalRulePriority=Speed  RndMeth=Simplest
  Constant : Constant  Value=0  SampleTime=-1
  Scope : Scope  NumInputPorts=3
  Scope1 : Scope  NumInputPorts=3
  Sum : Sum  Inputs=|++
  v>0 : Switch  Criteria=u2 > Threshold  Threshold=0.1  SaturateOnIntegerOverflow=off  InputSameDT=off
  TqRequest : Outport  VectorParamsAs1DForOutWhenUnconnected=off
  wires:
  AccPedal [0,1]/1 -> Scope/1, Acceleration Pedal Characteristic/1
  BrakePedal [0,1]/1 -> Scope/2, Brake Pedal Characteristic/1
  Acceleration Pedal Characteristic/1 -> Scope1/1, Sum/1
  Sum/1 -> Scope1/3, TqRequest/1
  Brake Pedal Characteristic/1 -> v>0/1
  Constant/1 -> v>0/3
  v>0/1 -> Scope1/2, Sum/2
  v [km/h]/1 -> v>0/2, Scope/3

== system Design_of_an_Energy_Efficient_Hybrid_Electric_Vehicle/All-Terrain Vehicle Model/Brake Torque/Smooth Sign ==
  1 : fl_lib/Physical Signals/Sources/PS Constant  constant=1
  2 : fl_ps_legacy_lib/Legacy Physical Signals/Functions/PS Gain  gain=2
  exp(2x) : fl_ps_legacy_lib/Legacy Physical Signals/Functions/PS Math Function  fcn_choice=3
      settings: InternalSimscapePortConfiguration="{\"Bottom\":[],\"Left\":[{\"id\":\"I\",\"label\":\"\",\"type\":\"input\"}],\"Right\":[{\"id\":\"O\",\"label\":\"\",\"type\":\"output\"}],\"Top\":[]}"
  exp(2x)+1 : fl_ps_legacy_lib/Legacy Physical Signals/Functions/PS Add
      settings: InternalSimscapePortConfiguration="{\"Bottom\":[],\"Left\":[{\"id\":\"I1\",\"label\":\"\",\"type\":\"input\"},{\"id\":\"I2\",\"label\":\"\",\"type\":\"input\"}],\"Right\":[{\"id\":\"O\",\"label\":\"\",\"type\":\"output\"}],\"Top\":[]}"
  exp(2x)-1 : fl_ps_legacy_lib/Legacy Physical Signals/Functions/PS Subtract
  tanh(x) : fl_ps_legacy_lib/Legacy Physical Signals/Functions/PS Divide
      settings: InternalSimscapePortConfiguration="{\"Bottom\":[],\"Left\":[{\"id\":\"I1\",\"label\":\"\",\"type\":\"input\"},{\"id\":\"I2\",\"label\":\"\",\"type\":\"input\"}],\"Right\":[{\"id\":\"O\",\"label\":\"\",\"type\":\"output\"}],\"Top\":[]}"
  x : PMIOPort  Side=Left
  y : PMIOPort  Port=2  Side=Right
  connections:
  y/RConn1 -- tanh(x)/RConn1
  x/RConn1 -- 2/LConn1
  exp(2x)-1/RConn1 -- tanh(x)/LConn1
  exp(2x)+1/RConn1 -- tanh(x)/LConn2
  exp(2x)+1/LConn2 -- exp(2x)-1/LConn1 -- exp(2x)/RConn1
  2/RConn1 -- exp(2x)/LConn1
  exp(2x)-1/LConn2 -- exp(2x)+1/LConn1 -- 1/RConn1

== system Design_of_an_Energy_Efficient_Hybrid_Electric_Vehicle/FOC/Alpha&Beta Current Estimation/Alpha_Beta_Estimation ==
  Idq_ref : Inport
  Theta : Inport  Port=2
  Add : Sum
  Add1 : Sum  Inputs=+-
  Demux : Demux  Outputs=2
  Fcn : Fcn  Expr=sin(u)
  Fcn1 : Fcn  Expr=cos(u)
  Gain : Gain
  Memory : Memory  InheritSampleTime=on
  Product{,1..3} (4 alike) : Product
  Scope : Scope
  Scope1 : Scope  NumInputPorts=2
  Sine-Cosine Lookup : mcbcontrolslib/Sine-Cosine Lookup  Commented=on  AngleInput=Radians  N_points=1024
  Ialpha_est : Outport
  Ibeta_est : Outport  Port=2
  wires:
  Idq_ref/1 -> Demux/1
  Demux/1 -> Product1/2, Product/2  "Id*"
  Demux/2 -> Product2/2, Product3/2  "Iq*"
  Product3/1 -> Add1/2
  Product/1 -> Add1/1
  Add1/1 -> Scope1/2, Ialpha_est/1  "Ialpha_est"
  Product1/1 -> Add/1
  Product2/1 -> Add/2
  Add/1 -> Ibeta_est/1, Scope1/1  "Ibeta_est"
  Gain/1 -> Memory/1, Scope/1
  Theta/1 -> Gain/1
  Fcn/1 -> Product3/1, Product1/1
  Fcn1/1 -> Product/1, Product2/1
  Memory/1 -> Fcn1/1, Fcn/1

== system Design_of_an_Energy_Efficient_Hybrid_Electric_Vehicle/FOC/Alpha&Beta Current Estimation/Transfrom_Alpha_Beta_Estimation ==
  Idq_ref : Inport
  theta : Inport  Port=2
  Add : Sum
  Add1 : Sum  Inputs=+-
  Add2 : Sum  Inputs=+-
  Constant1 : Constant  Value=(2*pi)/3  OutDataTypeStr=single  SampleTime=-1
  Demux : Demux  Outputs=2
  Fcn : Fcn  Expr=sin(u)
  Fcn1 : Fcn  Expr=cos(u)
  Gain : Gain
  Memory : Memory  InheritSampleTime=on
  Product{,1..3} (4 alike) : Product
  Scope : Scope
  "Ialpha\"_est" : Outport
  "Ibeta\"_est" : Outport  Port=2
  wires:
  Idq_ref/1 -> Demux/1
  Demux/1 -> Product1/2, Product/2  "Id*"
  Demux/2 -> Product2/2, Product3/2  "Iq*"
  Fcn1/1 -> Product/1, Product2/1
  Fcn/1 -> Product3/1, Product1/1
  Product3/1 -> Add1/2
  Product/1 -> Add1/1
  Add1/1 -> "Ialpha\"_est"/1  "Ialpha_est"
  Product1/1 -> Add/1
  Product2/1 -> Add/2
  Add/1 -> "Ibeta\"_est"/1  "Ibeta_est"
  theta/1 -> Gain/1
  Constant1/1 -> Add2/2
  Memory/1 -> Fcn1/1, Fcn/1
  Gain/1 -> Add2/1
  Add2/1 -> Scope/1, Memory/1

== system Design_of_an_Energy_Efficient_Hybrid_Electric_Vehicle/FOC/Speed Regulator1/Calculate position and speed ==
  VI_fb : Inport
  Demux : Demux  Outputs=2
  Scope : Scope  Commented=on  NumInputPorts=2
  Sliding Mode Observer : Subsystem
  Sliding Mode Observer (SMO) : Subsystem  Commented=on  mask(Sliding Mode Observer){Rs=pmsm.Rs, Ls=pmsm.Ld, MaxStatorVoltage=PU_System.V_base, MaxStatorCurrent=PU_System.I_base, Kslide=.1, E0=3, fo=360, Ts=Ts, SMO_params6=7, SMO_params7=2}
      mask prompts: Rs "Stator Resistance"; Ls "Stator Inductance"; MaxStatorVoltage "Maximum Stator Voltage"; MaxStatorCurrent "Maximum Stator Current"; Kslide "Sliding Control Gain"; E0 "Sliding Limit"; fo "filter_cutoff_frequency"; Ts "Block Sample Time"; SMO_params6 "Speed_Loop_Delay"; SMO_params7 "Spped_Loop_to_PU_Scaler"
      mask help: Created by Sankhadip Saha & Dipayan Saha
      mask TypeOptions SMO_params6: Debounce/Speed Loop Delay/DelayLength
      mask TypeOptions SMO_params7: Debounce/Speed_loop_to_PU_scaler/Gain
  Pos_PU : Outport
  speed_PU : Outport  Port=2
  wires:
  VI_fb/1 -> Sliding Mode Observer/1(InputSignals)
  Demux/1 -> Pos_PU/1
  Demux/2 -> speed_PU/1
  Sliding Mode Observer/1(Position/Speed) -> Demux/1
  Sliding Mode Observer (SMO)/1(Theta) -> Scope/1  "mySMO_θ"
  Sliding Mode Observer (SMO)/2(speed) -> Scope/2  "mySMO_w"
